simulink model "S5_Elevator_Position_Controller_Working_2016-12-08"  (R2014b)
settings: Solver=ode5  StartTime=0.0  StopTime=S  FixedStep=T  RelTol=1e-3
undefined symbols (not defined in the file or in its folder): Serial_Port, Standard_Devices, T
libraries: rapcon x4, simulink x1
settings Model: ModifiedByFormat=C. Gokcek  SimulationMode=external  ExtModeTrigDuration=50000  Creator=C. Gokcek  LastModifiedBy=C. Gokcek
settings DataIOCC: LimitDataPoints=off  SignalLoggingSaveFormat=ModelDataLogs  SaveOutput=off  SignalLogging=off  SaveTime=off
settings OptimizationCC: ExpressionDepthLimit=2147483647  InitFltsAndDblsToZero=on  SimCompilerOptimization=On
settings DebuggingCC: UnderspecifiedInitializationDetection=Classic  MergeDetectMultiDrivingBlocksExec=none  SolverPrmCheckMsg=none  ParameterPrecisionLossMsg=none  FcnCallInpInsideContextMsg=UseLocalSettings  StateNameClashWarn=warning
settings HardwareCC: ProdIntDivRoundTo=Zero  ProdEndianess=LittleEndian  ProdHWDeviceType=Intel->x86/Pentium  TargetIntDivRoundTo=Zero  TargetEndianess=LittleEndian  TargetHWDeviceType=Intel->x86/Pentium
settings RTWCC: SystemTargetFile=rtwin.tlc  TemplateMakefile=rtwin.tmf  Description=Real-Time Windows Target  RTWVerbose=off  TLCAssert=on  ProcessScript=rtwin_make_rtw_hook
settings CodeAppCC: GenerateComments=off  MaxIdLength=95  SimulinkBlockComments=off
settings RTWinTargetCC: TargetLibSuffix=_rtwin.lib  TargetPreCompLibLocation=C:\Program Files\MATLAB\R2014b\toolbox\rtw\targets\rtwin\lib\win64  ModelReferenceCompliant=off  CompOptLevelCompliant=off

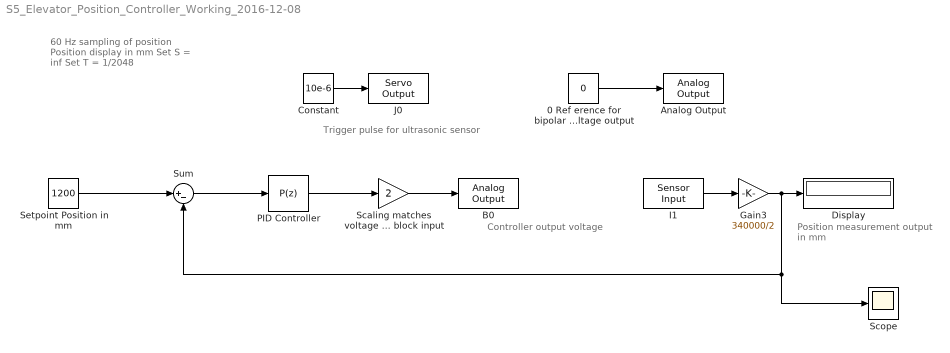
== system S5_Elevator_Position_Controller_Working_2016-12-08 ==
  note: Controller output
      | voltage
  note: Position measurement
      | output in mm
  note: Trigger pulse for ultrasonic sensor
  note: 60 Hz sampling of position
      | Position display in mm
      | Set S = inf
      | Set T = 1/2048
  0 Ref erence for bipolar voltage output : Constant  Value=0
  Analog Output : rapcon/Analog Output  SampleTime=T  MaxMissedTicks=10  ShowMissedTicks=0  YieldWhenWaiting=0  DrvName=Standard_Devices/Serial_Port  DrvAddress=5  DrvOptions=[460800 8 0 0 0 0 0 0]  PacketSize=8  DataTypes='double'  ShowReady=0  ShowError=0  PacketID=1  ByteOrder=1  InitialValue=0  FinalValue=0  CfgPrm=B0  PrmCfg=bipolar  ResVar=0  VarRes=0
  B0 : rapcon/Analog Output  SampleTime=T  MaxMissedTicks=10  ShowMissedTicks=0  YieldWhenWaiting=0  DrvName=Standard_Devices/Serial_Port  DrvAddress=5  DrvOptions=[460800 8 0 0 0 0 0 0]  PacketSize=8  DataTypes='double'  ShowReady=0  ShowError=0  PacketID=1  ByteOrder=1  InitialValue=0  FinalValue=0  CfgPrm=B1  PrmCfg=bipolar  ResVar=0  VarRes=0
  Constant : Constant  Value=10e-6  SampleTime=T
  Display : Display
  Gain3 : Gain  Gain=340000/2  OutDataTypeStr=double  SampleTime=T
  I1 : rapcon/Sensor Input  SampleTime=T  MaxMissedTicks=10  ShowMissedTicks=0  YieldWhenWaiting=0  DrvName=Standard_Devices/Serial_Port  DrvAddress=5  DrvOptions=[460800 8 0 0 0 0 0 0]  PacketSize=8  DataTypes='double'  ShowReady=0  ShowError=0  PacketID=1  ByteOrder=1  ShowTimestamp=0  CfgPrm=I1  PrmCfg=width  ResVar=0  VarRes=50
  J0 : rapcon/Servo Output  SampleTime=T  MaxMissedTicks=10  ShowMissedTicks=0  YieldWhenWaiting=0  DrvName=Standard_Devices/Serial_Port  DrvAddress=5  DrvOptions=[460800 8 0 0 0 0 0 0]  PacketSize=8  DataTypes='double'  ShowReady=0  ShowError=0  PacketID=1  ByteOrder=1  InitialValue=0  FinalValue=0  CfgPrm=J0  PrmCfg=width  ResVar=0  VarRes=50
  PID Controller : simulink/Continuous/PID Controller  Controller=P  TimeDomain=Discrete-time  SampleTime=T  IntegratorMethod=Forward Euler  FilterMethod=Forward Euler  Form=Parallel  P=.001992  I=.00001784  D=0  N=100  InitialConditionSource=internal  InitialConditionForIntegrator=0  InitialConditionForFilter=0  ExternalReset=none  LimitOutput=on  UpperSaturationLimit=16  LowerSaturationLimit=-16  LinearizeAsGain=on  AntiWindupMode=none  Kb=1  TrackingMode=off  Kt=1  PParamMin=[]  PParamMax=[]  IParamMin=[]  IParamMax=[]  DParamMin=[]  DParamMax=[]  NParamMin=[]  NParamMax=[]  KbParamMin=[]  KbParamMax=[]  KtParamMin=[]  KtParamMax=[]  POutMin=[]  POutMax=[]  IOutMin=[]  IOutMax=[]  DOutMin=[]  DOutMax=[]  NOutMin=[]  NOutMax=[]  KbOutMin=[]  KbOutMax=[]  KtOutMin=[]  KtOutMax=[]  IntegratorOutMin=[]  IntegratorOutMax=[]  FilterOutMin=[]  FilterOutMax=[]  SumOutMin=[]  SumOutMax=[]  SumI1OutMin=[]  SumI1OutMax=[]  SumI2OutMin=[]  SumI2OutMax=[]  SumI3OutMin=[]  SumI3OutMax=[]  SumDOutMin=[]  SumDOutMax=[]  SaturationOutMin=[]  SaturationOutMax=[]  IntegratorContinuousStateAttributes=''  IntegratorStateMustResolveToSignalObject=off  IntegratorRTWStateStorageClass=Auto  FilterContinuousStateAttributes=''  FilterStateMustResolveToSignalObject=off  FilterRTWStateStorageClass=Auto  DifferentiatorICPrevScaledInput=0  DifferentiatorOutMin=[]  DifferentiatorOutMax=[]  UseFilter=on
  "Scaling matches voltage applied to motor to block input " : Gain  Gain=2  SampleTime=T
  Scope : Scope
      settings: YMin=0  YMax=1500  ScrollMode=on
  Setpoint Position in mm : Constant  Value=1200  OutDataTypeStr=double  SampleTime=T
  Sum : Sum  Inputs=|+-
  wires:
  Gain3/1 -> Sum/2, Scope/1, Display/1
  I1/1 -> Gain3/1
  Constant/1 -> J0/1
  PID Controller/1 -> "Scaling matches voltage applied to motor to block input "/1
  0 Ref erence for bipolar voltage output/1 -> Analog Output/1
  "Scaling matches voltage applied to motor to block input "/1 -> B0/1
  Setpoint Position in mm/1 -> Sum/1
  Sum/1 -> PID Controller/1
